simulink model "simplifiedModel"  (R2025b)
settings: Solver=VariableStepAuto  StartTime=0.0  StopTime=30  RelTol=1e-3
undefined symbols (not defined in the file or in its folder): aRef, CR_AR, CR_mC, CR_Plan, CR_pos, dRef, NFins, rocketLength, rT, SF_aFin, SF_AR, SF_CG, SF_CP_Sub, SF_CP_sup, SF_H, SF_mC, SF_plan, SF_RC, SF_TC, yMac
libraries: aerolibasang x3, aerolibanim x2, simulink_extras x1, aerolibatmos2 x1
settings Model: Creator=Ranvir  LastModifiedBy=Ranvir

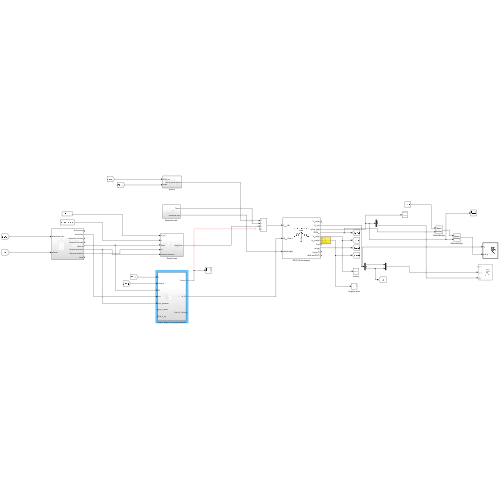
[thumbnail: Simulink's stored preview of the top-level diagram]
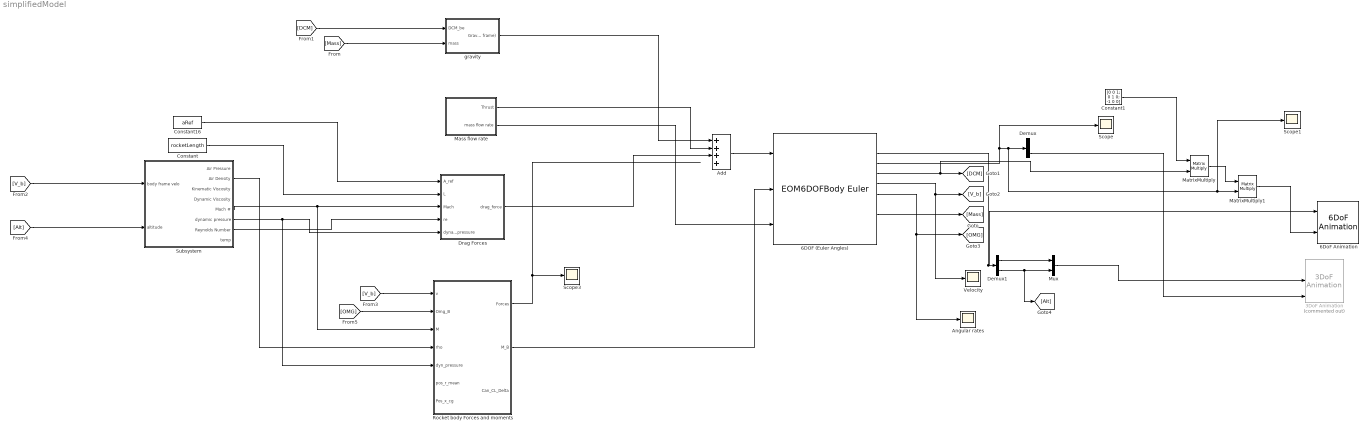
== system simplifiedModel ==
  3DoF Animation : aerolibanim/3DoF Animation  Commented=on  u1=[0 5000 -2000 2000 -5050 -3050]  u2=0.05  u3=10  u5=Fixed position  u6=[2000 500 -3150]  u7=10  u8=on
  6DOF (Euler Angles) : EOM6DOFBodyEuler  mtype=Simple Variable  eul_0=[0 deg2rad(5) 0]  mass_0=23.434  mass_e=16.5  mass_f=23.434  inertia_e=[9.947 0 0; 0 9.947 0; 0 0 0.14158]  inertia_f=[14.126568 0 0; 0 14.126568 0; 0 0 0.201075]  mass_flag=on
  6DoF Animation : aerolibanim/6DoF Animation  u1=[0 4000 -2000 2000 -5000 -3000]  u2=0.01  u3=100  u4=[4000 0 -5000]  u5=Fly alongside  u6=[2000 500 -3150]  u7=2  u8=off
  Add : Sum  Inputs=++++
  Angular rates : Scope
      settings: ActiveDisplayYMinimum=-0.094477943134186726  ActiveDisplayYMaximum=0.85030148820768081  DataLoggingVariableName=ScopeData8
  Constant : Constant  Value=rocketLength
  Constant1 : Constant  Value=[0 0 1; 0 1 0; -1 0 0]
  Constant16 : Constant  Value=aRef
  Demux : Demux  Outputs=3
  Demux1 : Demux  Outputs=3
  Drag Forces : Subsystem
  Mass flow rate : Subsystem
  MatrixMultiply : Product  Multiplication=Matrix(*)
  MatrixMultiply1 : Product  Multiplication=Matrix(*)
  Mux : Mux  Inputs=2
  Rocket body Forces and moments : Subsystem
  Scope : Scope
      settings: ActiveDisplayYMinimum=-3.9094785431209607  ActiveDisplayYMaximum=3.92160420988626
  Scope1 : Scope
      settings: ActiveDisplayYMinimum=-1  ActiveDisplayYMaximum=1  DataLoggingVariableName=ScopeData2
  Scope3 : Scope
      settings: ActiveDisplayYMinimum=-1.6641307477969988E+6  ActiveDisplayYMaximum=1.5617591567603932E+6  DataLoggingVariableName=ScopeData10
  Subsystem : Subsystem
  Velocity : Scope
      settings: ActiveDisplayYMinimum=-80.5453519654905  ActiveDisplayYMaximum=285.45576994763  DataLoggingVariableName=ScopeData11
  gravity : Subsystem
  wires:
  Subsystem/5(Mach #) -> Drag Forces/3(Mach), Rocket body Forces and moments/3(M)
  Subsystem/7(Reynolds Number) -> Drag Forces/4(re)
  Subsystem/6(dynamic pressure) -> Rocket body Forces and moments/5(dyn_pressure), Drag Forces/5(dynamic pressure)
  Constant16/1 -> Drag Forces/1(A_ref)
  Constant/1 -> Drag Forces/2(L)
  Mass flow rate/1(Thrust) -> Add/2
  gravity/1(Gravity (body frame)) -> Add/1
  Mass flow rate/2(mass flow rate) -> 6DOF (Euler Angles)/3
  6DOF (Euler Angles)/8 -> [Mass]
  [Mass] -> gravity/2(mass)
  6DOF (Euler Angles)/4 -> MatrixMultiply/2, [DCM]
  [DCM] -> gravity/1(DCM_be)
  Add/1 -> 6DOF (Euler Angles)/1
  Drag Forces/1(drag_force) -> Add/3
  Rocket body Forces and moments/2(M_B) -> 6DOF (Euler Angles)/2
  6DOF (Euler Angles)/3 -> Scope/1, Scope1/1, MatrixMultiply1/2, Demux/1
  6DOF (Euler Angles)/2 -> 6DoF Animation/1, Demux1/1
  Demux1/1 -> Mux/1
  Demux1/3 -> [Alt], Mux/2
  Mux/1 -> 3DoF Animation/2
  6DOF (Euler Angles)/5 -> Velocity/1, [V_b]
  [V_b] -> Subsystem/1(body frame velo)
  [V_b] -> Rocket body Forces and moments/1(v)
  6DOF (Euler Angles)/6 -> Angular rates/1, [OMG]
  [Alt] -> Subsystem/2(altitude)
  [OMG] -> Rocket body Forces and moments/2(Omg_B)
  Subsystem/2(Air Density) -> Rocket body Forces and moments/4(rho)
  Demux/3 -> 3DoF Animation/3
  Constant1/1 -> MatrixMultiply/1
  MatrixMultiply/1 -> MatrixMultiply1/1
  MatrixMultiply1/1 -> 6DoF Animation/2
  Rocket body Forces and moments/1(Forces) -> Scope3/1

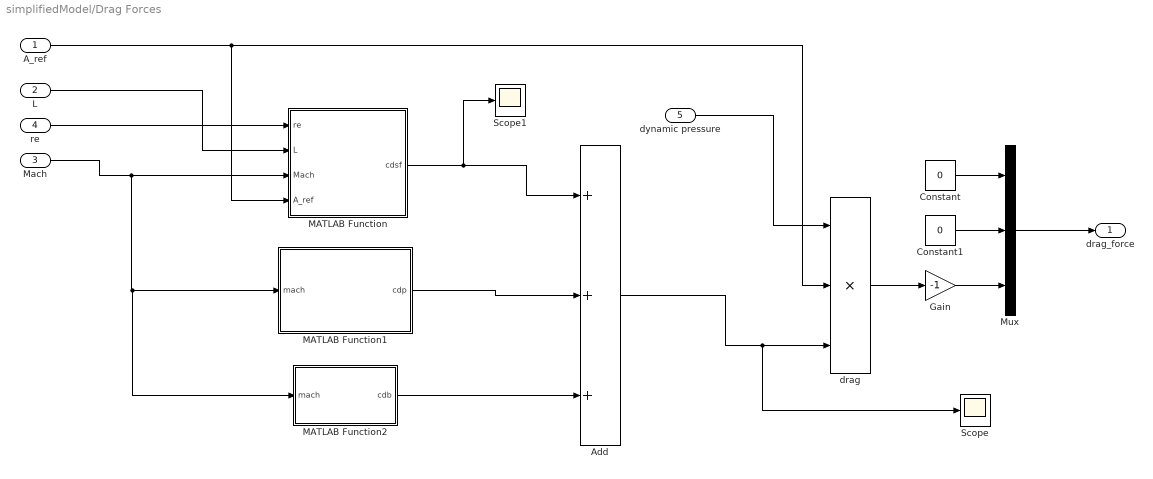
== system simplifiedModel/Drag Forces ==
  A_ref : Inport
  L : Inport  Port=2
  Mach : Inport  Port=3
  re : Inport  Port=4
  dynamic pressure : Inport  Port=5
  Add : Sum  Inputs=+++
  Constant : Constant  Value=0
  Constant1 : Constant  Value=0
  Gain : Gain  Gain=-1
  MATLAB Function : MATLAB Function  TreatAsAtomicUnit=on
  MATLAB Function1 : MATLAB Function  TreatAsAtomicUnit=on
  MATLAB Function2 : MATLAB Function  TreatAsAtomicUnit=on
  Mux : Mux  Inputs=3
  Scope : Scope
      settings: ActiveDisplayYMinimum=0.21944409933855474  ActiveDisplayYMaximum=1.41457657842317  DataLoggingVariableName=ScopeData7
  Scope1 : Scope
      settings: ActiveDisplayYMinimum=0.20880537476084277  ActiveDisplayYMaximum=1.0462233981932223  DataLoggingVariableName=ScopeData9
  drag : Product  Inputs=3
  drag_force : Outport
  wires:
  L/1 -> MATLAB Function/2(L)
  A_ref/1 -> drag/2, MATLAB Function/4(A_ref)
  Mach/1 -> MATLAB Function2/1(mach), MATLAB Function1/1(mach), MATLAB Function/3(Mach)
  re/1 -> MATLAB Function/1(re)
  MATLAB Function2/1(cdb) -> Add/3
  MATLAB Function1/1(cdp) -> Add/2
  MATLAB Function/1(cdsf) -> Scope1/1, Add/1
  dynamic pressure/1 -> drag/1
  Add/1 -> Scope/1, drag/3
  drag/1 -> Gain/1
  Mux/1 -> drag_force/1
  Constant1/1 -> Mux/2
  Gain/1 -> Mux/3
  Constant/1 -> Mux/1

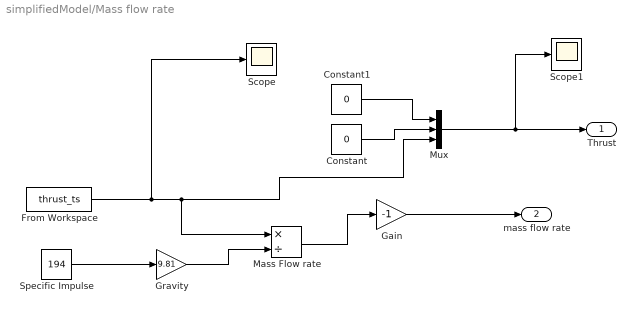
== system simplifiedModel/Mass flow rate ==
  Constant : Constant  Value=0
  Constant1 : Constant  Value=0
  From Workspace : FromWorkspace  VariableName=thrust_ts  OutputAfterFinalValue=Setting to zero
  Gain : Gain  Gain=-1
  Gravity : Gain  Gain=9.81
  Mass Flow rate : Product  Inputs=*/
  Mux : Mux  Inputs=3
  Scope : Scope
      settings: DataLoggingVariableName=ScopeData6
  Scope1 : Scope
      settings: ActiveDisplayYMinimum=-1  ActiveDisplayYMaximum=1
  Specific Impulse : Constant  Value=194
  Thrust : Outport
  mass flow rate : Outport  Port=2
  wires:
  Mass Flow rate/1 -> Gain/1
  Gravity/1 -> Mass Flow rate/2
  Specific Impulse/1 -> Gravity/1
  From Workspace/1 -> Scope/1, Mux/3, Mass Flow rate/1
  Gain/1 -> mass flow rate/1
  Constant/1 -> Mux/2
  Constant1/1 -> Mux/1
  Mux/1 -> Scope1/1, Thrust/1

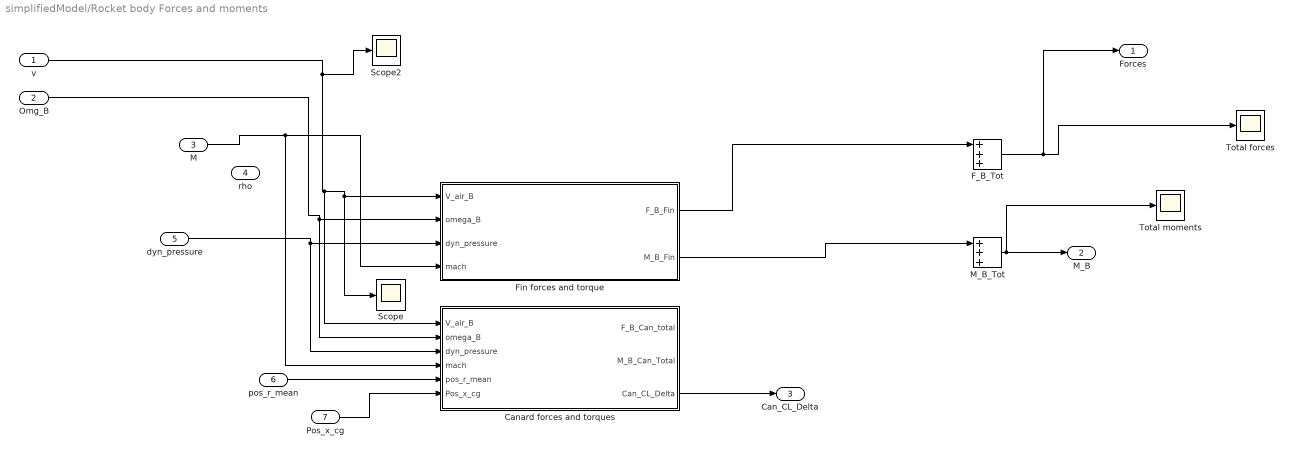
== system simplifiedModel/Rocket body Forces and moments ==
  v : Inport
  Omg_B : Inport  Port=2
  M : Inport  Port=3
  rho : Inport  Port=4
  dyn_pressure : Inport  Port=5
  pos_r_mean : Inport  Port=6
  Pos_x_cg : Inport  Port=7
  Canard forces and torques : Subsystem
  F_B_Tot : Sum  Inputs=+++
  Fin forces and torque : Subsystem
  M_B_Tot : Sum  Inputs=+++
  Scope : Scope
      settings: ActiveDisplayYMinimum=-0.018508285271356052  ActiveDisplayYMaximum=0.020281407753936571  DataLoggingVariableName=ScopeData15
  Scope2 : Scope
      settings: ActiveDisplayYMinimum=-769.59974570590657  ActiveDisplayYMaximum=2344.982620265816  DataLoggingVariableName=ScopeData16
  Total forces : Scope
      settings: ActiveDisplayYMinimum=-5.1479877420967748  ActiveDisplayYMaximum=7.0544525068547062  DataLoggingVariableName=ScopeData19
  Total moments : Scope
      settings: ActiveDisplayYMinimum=-0.69221418098949072  ActiveDisplayYMaximum=0.72914847927075177  DataLoggingVariableName=ScopeData17
  Forces : Outport
  M_B : Outport  Port=2
  Can_CL_Delta : Outport  Port=3
  wires:
  Fin forces and torque/1(F_B_Fin) -> F_B_Tot/1
  M_B_Tot/1 -> Total moments/1, M_B/1
  Canard forces and torques/3(Can_CL_Delta) -> Can_CL_Delta/1
  F_B_Tot/1 -> Forces/1, Total forces/1
  v/1 -> Canard forces and torques/1(V_air_B), Scope/1, Fin forces and torque/1(V_air_B), Scope2/1
  Omg_B/1 -> Canard forces and torques/2(omega_B), Fin forces and torque/2(omega_B)
  M/1 -> Canard forces and torques/4(mach), Fin forces and torque/4(mach)
  dyn_pressure/1 -> Canard forces and torques/3(dyn_pressure), Fin forces and torque/3(dyn_pressure)
  pos_r_mean/1 -> Canard forces and torques/5(pos_r_mean)
  Pos_x_cg/1 -> Canard forces and torques/6(Pos_x_cg)
  Fin forces and torque/2(M_B_Fin) -> M_B_Tot/1

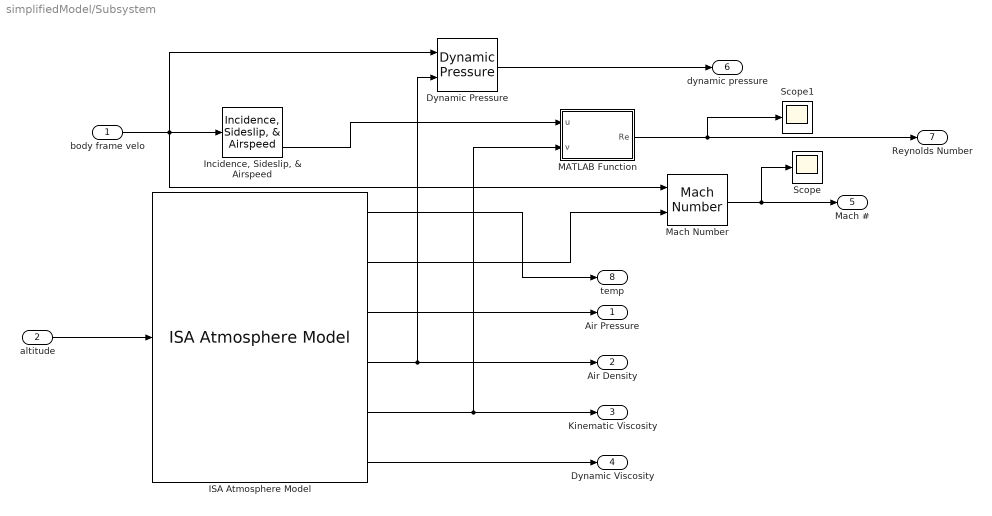
== system simplifiedModel/Subsystem ==
  body frame velo : Inport
  altitude : Inport  Port=2
  Dynamic Pressure : aerolibasang/Dynamic Pressure
  ISA Atmosphere Model : aerolibatmos2/ISA Atmosphere Model  useExtended=off  action=None  custom=off  viscosityOut=on  g=9.80665  gamma=1.4  R=287.0531  L=0.0065  h_trop=11000  h_strat=20000  rho0=1.225  P0=101325  T0=288.15  h0=0  S=110.4  Tref=273.15  muref=1.716e-5
  "Incidence, Sideslip, & Airspeed" : aerolibasang/Incidence, Sideslip, & Airspeed
  MATLAB Function : MATLAB Function  TreatAsAtomicUnit=on
  Mach Number : aerolibasang/Mach Number
  Scope : Scope
      settings: ActiveDisplayYMinimum=-1  ActiveDisplayYMaximum=1  DataLoggingVariableName=ScopeData4
  Scope1 : Scope
      settings: ActiveDisplayYMinimum=-4.9384528358794907E+6  ActiveDisplayYMaximum=4.4446075522915423E+7  DataLoggingVariableName=ScopeData5
  Air Pressure : Outport
  Air Density : Outport  Port=2
  Kinematic Viscosity : Outport  Port=3
  Dynamic Viscosity : Outport  Port=4
  Mach # : Outport  Port=5
  dynamic pressure : Outport  Port=6
  Reynolds Number : Outport  Port=7
  temp : Outport  Port=8
  wires:
  ISA Atmosphere Model/2 -> Mach Number/2
  ISA Atmosphere Model/5 -> MATLAB Function/2(v), Kinematic Viscosity/1
  ISA Atmosphere Model/4 -> Dynamic Pressure/2, Air Density/1
  ISA Atmosphere Model/3 -> Air Pressure/1
  ISA Atmosphere Model/6 -> Dynamic Viscosity/1
  Mach Number/1 -> Scope/1, Mach #/1
  altitude/1 -> ISA Atmosphere Model/1
  Dynamic Pressure/1 -> dynamic pressure/1
  body frame velo/1 -> Dynamic Pressure/1, Mach Number/1, "Incidence, Sideslip, & Airspeed"/1
  "Incidence, Sideslip, & Airspeed"/3 -> MATLAB Function/1(u)
  MATLAB Function/1(Re) -> Reynolds Number/1, Scope1/1
  ISA Atmosphere Model/1 -> temp/1

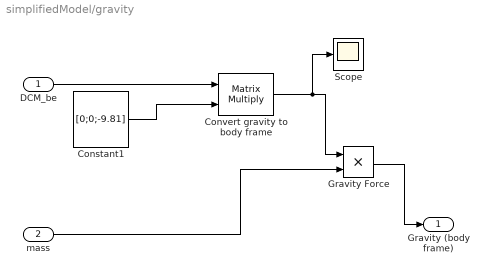
== system simplifiedModel/gravity ==
  DCM_be : Inport
  mass : Inport  Port=2
  Constant1 : Constant  Value=[0;0;-9.81]  VectorParams1D=off
  Convert gravity to body frame : Product  Multiplication=Matrix(*)
  Gravity Force : Product
  Scope : Scope
      settings: ActiveDisplayYMinimum=-1  ActiveDisplayYMaximum=1  DataLoggingVariableName=ScopeData3
  Gravity (body frame) : Outport
  wires:
  mass/1 -> Gravity Force/2
  Gravity Force/1 -> Gravity (body frame)/1
  Constant1/1 -> Convert gravity to body frame/2
  DCM_be/1 -> Convert gravity to body frame/1
  Convert gravity to body frame/1 -> Scope/1, Gravity Force/1

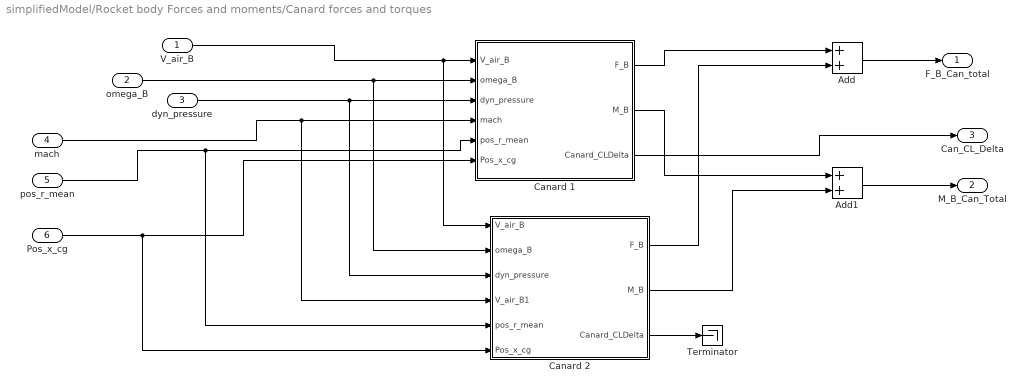
== system simplifiedModel/Rocket body Forces and moments/Canard forces and torques ==
  V_air_B : Inport
  omega_B : Inport  Port=2
  dyn_pressure : Inport  Port=3
  mach : Inport  Port=4
  pos_r_mean : Inport  Port=5
  Pos_x_cg : Inport  Port=6
  Add : Sum
  Add1 : Sum
  Canard 1 : Subsystem
  Canard 2 : Subsystem
  Terminator : Terminator
  F_B_Can_total : Outport
  M_B_Can_Total : Outport  Port=2
  Can_CL_Delta : Outport  Port=3
  wires:
  Canard 1/1(F_B) -> Add/1
  Canard 2/1(F_B) -> Add/2
  Canard 1/2(M_B) -> Add1/1
  Canard 2/2(M_B) -> Add1/2
  Add/1 -> F_B_Can_total/1
  Add1/1 -> M_B_Can_Total/1
  Canard 1/3(Canard_CLDelta) -> Can_CL_Delta/1
  Canard 2/3(Canard_CLDelta) -> Terminator/1
  V_air_B/1 -> Canard 2/1(V_air_B), Canard 1/1(V_air_B)
  omega_B/1 -> Canard 2/2(omega_B), Canard 1/2(omega_B)
  dyn_pressure/1 -> Canard 2/3(dyn_pressure), Canard 1/3(dyn_pressure)
  mach/1 -> Canard 2/4(V_air_B1), Canard 1/4(mach)
  pos_r_mean/1 -> Canard 2/5(pos_r_mean), Canard 1/5(pos_r_mean)
  Pos_x_cg/1 -> Canard 2/6(Pos_x_cg), Canard 1/6(Pos_x_cg)

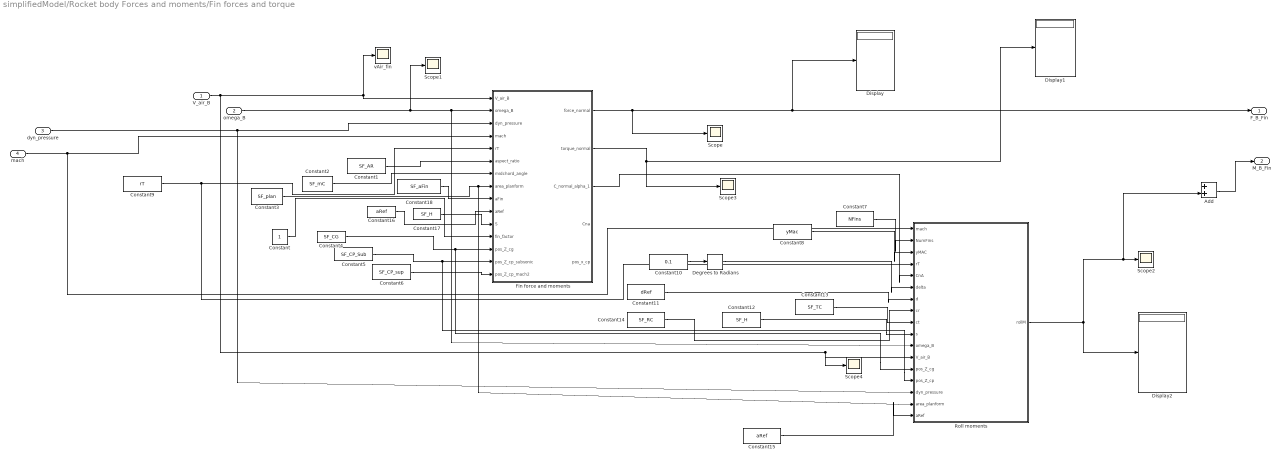
== system simplifiedModel/Rocket body Forces and moments/Fin forces and torque ==
  V_air_B : Inport
  omega_B : Inport  Port=2
  dyn_pressure : Inport  Port=3
  mach : Inport  Port=4
  Add : Sum
  Constant : Constant
  Constant1 : Constant  Value=SF_AR
  Constant10 : Constant  Value=0.1
  Constant11 : Constant  Value=dRef
  Constant12 : Constant  Value=SF_H
  Constant13 : Constant  Value=SF_TC
  Constant14 : Constant  Value=SF_RC
  Constant15 : Constant  Value=aRef
  Constant16 : Constant  Value=aRef
  Constant17 : Constant  Value=SF_H
  Constant18 : Constant  Value=SF_aFin
  Constant2 : Constant  Value=SF_mC
  Constant3 : Constant  Value=SF_plan
  Constant4 : Constant  Value=SF_CG
  Constant5 : Constant  Value=SF_CP_Sub
  Constant6 : Constant  Value=SF_CP_sup
  Constant7 : Constant  Value=NFins
  Constant8 : Constant  Value=yMac
  Constant9 : Constant  Value=rT
  Degrees to Radians : simulink_extras/Transformations/Degrees to Radians
  Display : Display
  Display1 : Display
  Display2 : Display
  Fin force and moments : MATLAB Function  TreatAsAtomicUnit=on
  Roll moments : MATLAB Function  TreatAsAtomicUnit=on
  Scope{,1..4} (5 alike) : Scope
      Scope settings: ActiveDisplayYMinimum=-38.327533693921524  ActiveDisplayYMaximum=344.94780324529376  DataLoggingVariableName=ScopeData13
      Scope1 settings: ActiveDisplayYMinimum=-1  ActiveDisplayYMaximum=1  DataLoggingVariableName=ScopeData23
      Scope2 settings: ActiveDisplayYMinimum=-0.01388327582792423  ActiveDisplayYMaximum=0.055054556987143094  DataLoggingVariableName=ScopeData24
      Scope3 settings: ActiveDisplayYMinimum=-1  ActiveDisplayYMaximum=1  DataLoggingVariableName=ScopeData27
      Scope4 settings: ActiveDisplayYMinimum=-1  ActiveDisplayYMaximum=1  DataLoggingVariableName=ScopeData28
  vAir_fin : Scope
      settings: ActiveDisplayYMinimum=-80.543649923632159  ActiveDisplayYMaximum=285.44044964997647  DataLoggingVariableName=ScopeData14
  F_B_Fin : Outport
  M_B_Fin : Outport  Port=2
  wires:
  Fin force and moments/1(force_normal) -> Scope/1, Display/1, F_B_Fin/1
  Fin force and moments/2(torque_normal) -> Scope3/1, Display1/1
  Constant6/1 -> Fin force and moments/15(pos_Z_cp_mach2)
  Constant5/1 -> Roll moments/14(pos_Z_cp), Fin force and moments/14(pos_Z_cp_subsonic)
  Constant4/1 -> Roll moments/13(pos_Z_cg), Fin force and moments/13(pos_Z_cg)
  Constant/1 -> Fin force and moments/12(fin_factor)
  Constant3/1 -> Roll moments/16(area_planform), Fin force and moments/8(area_planform)
  Constant2/1 -> Fin force and moments/7(midchord_angle)
  Constant1/1 -> Fin force and moments/6(aspect_ratio)
  V_air_B/1 -> Scope4/1, Roll moments/12(V_air_B), vAir_fin/1, Fin force and moments/1(V_air_B)
  mach/1 -> Roll moments/1(mach), Fin force and moments/4(mach)
  dyn_pressure/1 -> Roll moments/15(dyn_pressure), Fin force and moments/3(dyn_pressure)
  omega_B/1 -> Roll moments/11(omega_B), Fin force and moments/2(omega_B), Scope1/1
  Constant7/1 -> Roll moments/2(NumFins)
  Constant11/1 -> Roll moments/7(d)
  Constant10/1 -> Degrees to Radians/1
  Constant9/1 -> Roll moments/4(rT), Fin force and moments/5(rT)
  Constant8/1 -> Roll moments/3(yMAC)
  Constant12/1 -> Roll moments/10(s)
  Constant13/1 -> Roll moments/9(ct)
  Constant14/1 -> Roll moments/8(cr)
  Roll moments/1(rollM) -> Add/2, Scope2/1, Display2/1
  Constant15/1 -> Roll moments/17(aRef)
  Constant16/1 -> Fin force and moments/10(aRef)
  Constant17/1 -> Fin force and moments/11(S)
  Constant18/1 -> Fin force and moments/9(aFin)
  Degrees to Radians/1 -> Roll moments/6(delta)
  Fin force and moments/3(C_normal_alpha_1) -> Roll moments/5(CnA)
  Add/1 -> M_B_Fin/1

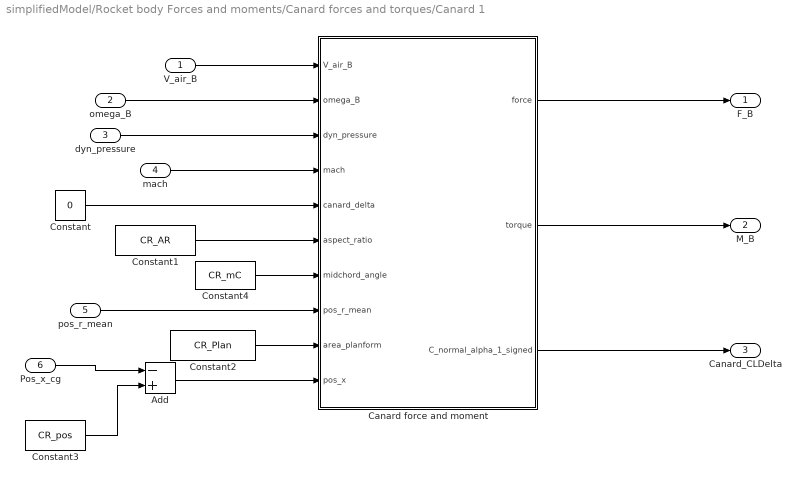
== system simplifiedModel/Rocket body Forces and moments/Canard forces and torques/Canard 1 ==
  V_air_B : Inport
  omega_B : Inport  Port=2
  dyn_pressure : Inport  Port=3
  mach : Inport  Port=4
  pos_r_mean : Inport  Port=5
  Pos_x_cg : Inport  Port=6
  Add : Sum  Inputs=-+
  Canard force and moment : MATLAB Function  TreatAsAtomicUnit=on
  Constant : Constant  Value=0
  Constant1 : Constant  Value=CR_AR
  Constant2 : Constant  Value=CR_Plan
  Constant3 : Constant  Value=CR_pos
  Constant4 : Constant  Value=CR_mC
  F_B : Outport
  M_B : Outport  Port=2
  Canard_CLDelta : Outport  Port=3
  wires:
  Canard force and moment/1(force) -> F_B/1
  Canard force and moment/2(torque) -> M_B/1
  Canard force and moment/3(C_normal_alpha_1_signed) -> Canard_CLDelta/1
  Constant/1 -> Canard force and moment/5(canard_delta)
  V_air_B/1 -> Canard force and moment/1(V_air_B)
  omega_B/1 -> Canard force and moment/2(omega_B)
  dyn_pressure/1 -> Canard force and moment/3(dyn_pressure)
  mach/1 -> Canard force and moment/4(mach)
  pos_r_mean/1 -> Canard force and moment/8(pos_r_mean)
  Pos_x_cg/1 -> Add/1
  Add/1 -> Canard force and moment/10(pos_x)
  Constant3/1 -> Add/2
  Constant2/1 -> Canard force and moment/9(area_planform)
  Constant1/1 -> Canard force and moment/6(aspect_ratio)
  Constant4/1 -> Canard force and moment/7(midchord_angle)

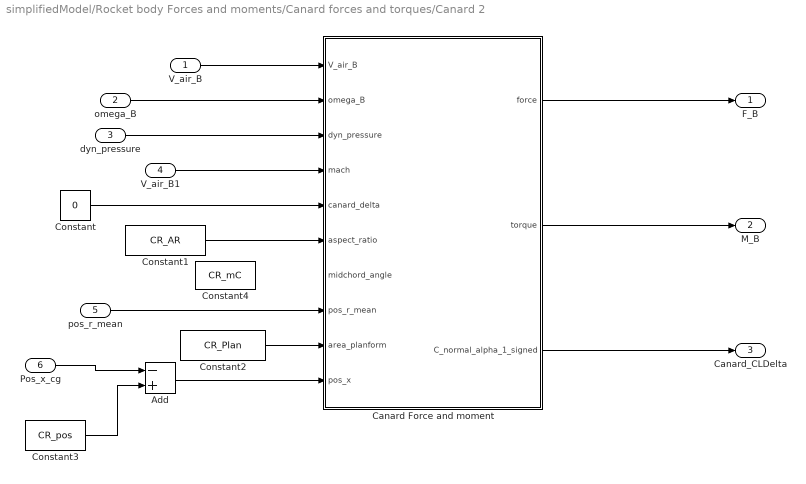
== system simplifiedModel/Rocket body Forces and moments/Canard forces and torques/Canard 2 ==
  V_air_B : Inport
  omega_B : Inport  Port=2
  dyn_pressure : Inport  Port=3
  V_air_B1 : Inport  Port=4
  pos_r_mean : Inport  Port=5
  Pos_x_cg : Inport  Port=6
  Add : Sum  Inputs=-+
  Canard Force and moment : MATLAB Function  TreatAsAtomicUnit=on
  Constant : Constant  Value=0
  Constant1 : Constant  Value=CR_AR
  Constant2 : Constant  Value=CR_Plan
  Constant3 : Constant  Value=CR_pos
  Constant4 : Constant  Value=CR_mC
  F_B : Outport
  M_B : Outport  Port=2
  Canard_CLDelta : Outport  Port=3
  wires:
  Canard Force and moment/1(force) -> F_B/1
  Canard Force and moment/2(torque) -> M_B/1
  Canard Force and moment/3(C_normal_alpha_1_signed) -> Canard_CLDelta/1
  V_air_B1/1 -> Canard Force and moment/4(mach)
  omega_B/1 -> Canard Force and moment/2(omega_B)
  Constant2/1 -> Canard Force and moment/9(area_planform)
  V_air_B/1 -> Canard Force and moment/1(V_air_B)
  dyn_pressure/1 -> Canard Force and moment/3(dyn_pressure)
  Constant/1 -> Canard Force and moment/5(canard_delta)
  Constant3/1 -> Add/2
  Pos_x_cg/1 -> Add/1
  Constant1/1 -> Canard Force and moment/6(aspect_ratio)
  pos_r_mean/1 -> Canard Force and moment/8(pos_r_mean)
  Add/1 -> Canard Force and moment/10(pos_x)

== matlab function simplifiedModel/Rocket body Forces and moments/Fin forces and torque/Roll moments ==
  data: mach input; NumFins input; rollM output; yMAC input; rT input; CnA input; delta input; d input; cr input; ct input; s input; omega_B input; V_air_B input; pos_Z_cg input; pos_Z_cp input; dyn_pressure input; area_planform input; aRef input
function rollM  = roll_moment(mach, NumFins, yMAC, rT, CnA, delta, d, cr, ct,s, omega_B, V_air_B, pos_Z_cg, pos_Z_cp, dyn_pressure, area_planform, aRef)
    



   
    pos_z = (pos_Z_cp - pos_Z_cg) * [0;0;1];
    
    % need to know incidence angle and how to convert vector into direciton
    %%% relative velocity


    %Define the vector using the wind vector, use that to create the moment
    %definition (z axis in the body frame) then multiply that with the 
    
    %%% relative velocity
    Vrel = V_air_B + cross(omega_B, pos_z);

    
    Vrel_Z = Vrel(3);
    Vrel_mag = norm(Vrel);
   
    beta = sqrt(abs(1-mach^2));
    cn_0 = (2*pi)/beta;


    rollForcing = (NumFins*(yMAC+rT)*CnA*delta)/s;
    %% Roll damping bs
    if Vrel(3) ~= 0
        %sumTerm = (((cr+ct)/2)*(rT^2)*s) + (((cr+(2*ct))/3)*(s^2)*rT) + (((cr+(3*ct))/12)*(s^3));
    
        %Fix from chatgpt
        sumTerm = ((cr+ct)/2)      * (rT^2) * s  + ...
          ((cr+2*ct)/3)    * (rT)   * (s^2) + ...
          ((cr+3*ct)/12)   * (s^3);

        rDampCoeff = ((NumFins*cn_0*omega_B(3))/(aRef*d*Vrel_mag))*sumTerm

    
            
        cRl = rollForcing - rDampCoeff;
    
        F_N_dir = [
                   0;
                   0;
                   Vrel_Z/Vrel_mag;
                  ];
        
         f_m = cRl * dyn_pressure * aRef*d;

         rollM = [0; 0; f_m;];
    else
        rollM =[0; 0; 0;];
 
    %rollM = cross(pos_z, force_normal);

end

== matlab function simplifiedModel/Rocket body Forces and moments/Canard forces and torques/Canard 1/Canard force and moment ==
  data: V_air_B input; force output; omega_B input; dyn_pressure input; mach input; canard_delta input; aspect_ratio input; midchord_angle input; pos_r_mean input; area_planform input; pos_x input; torque output; C_normal_alpha_1_signed output
function [force, torque, C_normal_alpha_1_signed] = canard_dynamics(V_air_B, omega_B, dyn_pressure, mach, canard_delta, aspect_ratio, midchord_angle, pos_r_mean, area_planform, pos_x)
    % canard position
    pos = [pos_x; pos_r_mean; 0];

    % relative velocity
    Vrel = V_air_B + cross(omega_B, pos);
    
    % local incidence 
    alpha_local = atan2(Vrel(3), Vrel(1));
    incidence = canard_delta - alpha_local;
    
    % calculate coefficient of planar surface
    C_normal_alpha_1 = aerosurface_calc(mach, incidence, aspect_ratio, midchord_angle);
    C_normal_alpha_1_signed = C_normal_alpha_1 * sign(Vrel(1));
    
    % force and torque
    force = C_normal_alpha_1 * area_planform * sin(incidence) * dyn_pressure * [0; 0; 1];
    torque = cross(pos, force);
end

== matlab function simplifiedModel/Drag Forces/MATLAB Function ==
  data: re input; L input; cdsf output; Mach input; A_ref input
function cdsf = skin_friction(re,L, Mach,A_ref)

r_s = 425e-6;

f_b = 8.93;
chord_mean = 0.23456;
t = 0.00686;

A_wetbody = 0.7009;
A_wetfin = 0.1609;

re_crit = 51*(r_s/L)^-1.039;

if re < 10^4
    cf = 1.48e-2;
elseif re >= 10^4 && re < re_crit
    cf = 1 / (1.5*log(re) - 5.6)^2;
else
    cf = 0.032*(r_s/L)^0.2;
end

if Mach < 1
    c_fc = cf*(1-0.1*Mach^2);
else 
    c_fc = cf/(1+0.15*Mach^2)^0.58;
end

cdsf = c_fc * (((1+(1/(2*f_b)))*A_wetbody + ((1+(2*t/chord_mean)))*A_wetfin)/A_ref);

== matlab function simplifiedModel/Subsystem/MATLAB Function ==
  data: u input; Re output; v input
function Re = reynolds(u,v)
L = 2.13;

Re = (u*L)/v;

== matlab function simplifiedModel/Drag Forces/MATLAB Function1 ==
  data: cdp output; mach input
function cdp = pressure_drag(mach)

sweep_angle = 1.13446;

if mach < 0.9
    cd_le = (1-mach^2)^(-0.417) - 1;
elseif mach>=0.9 && mach<1
   cd_le = 1-1.785*(mach-0.9);
else
    cd_le = 1.214-((0.502)/(mach^2))+((0.1095)/(mach^4));
end

cdp = cd_le * cos(sweep_angle)^2;

== matlab function simplifiedModel/Drag Forces/MATLAB Function2 ==
  data: mach input; cdb output
function cdb = base_drag(mach)

if mach < 1
    cdb = 0.12 + 0.13*mach^2;
else
    cdb = 0.25/mach;
end

== matlab function simplifiedModel/Rocket body Forces and moments/Fin forces and torque/Fin force and moments ==
  data: V_air_B input; force_normal output; omega_B input; dyn_pressure input; mach input; rT input; aspect_ratio input; midchord_angle input; area_planform input; aFin input; aRef input; S input; fin_factor input; pos_Z_cg input; pos_Z_cp_subsonic input; pos_Z_cp_mach2 input; torque_normal output; C_normal_alpha_1 output; Cna output; pos_x_cp output
function [force_normal, torque_normal, C_normal_alpha_1, Cna,  pos_x_cp] = fin_dynamics(V_air_B, omega_B, dyn_pressure, mach, rT, aspect_ratio, midchord_angle, area_planform, aFin, aRef, S, fin_factor, pos_Z_cg, pos_Z_cp_subsonic, pos_Z_cp_mach2)
 %%% Center of Pressure
    % threshold values
    subsonic = 0.8;
    supersonic = 1.6;

    % linear interpolation (for now)
    if mach <= subsonic
        pos_x_cp = pos_Z_cp_subsonic;
    elseif mach >= supersonic 
        pos_x_cp = pos_Z_cp_mach2;
    else % transonic
        pos_x_cp = (mach - supersonic) * (pos_Z_cp_subsonic - pos_Z_cp_mach2) / (subsonic - supersonic) + pos_Z_cp_mach2;
    end

    pos_z = (pos_x_cp - pos_Z_cg) * [0;0;1];

    
    %%% relative velocity
    Vrel = V_air_B + cross(omega_B, pos_z);

    % Body relative velocity magnitude
    Vrel_mag = norm(Vrel);
    Vrel_Z = Vrel(3);
    Vrel_magXY = norm(Vrel(1:2));
    incidence = atan2(Vrel_magXY,Vrel_Z);

    %%% calculate normal force coefficient
    C_normal_alpha_1 = aerosurface_calc(mach, incidence, aspect_ratio, midchord_angle)*(1+(rT/(S+rT)));
    
    Cna = (2*C_normal_alpha_1);
    %%% Forces
    if Vrel_magXY ~= 0 % prevent division by 0
        % Angle of attack and component separation
        
        F_N_dir = [
                   Vrel(1) / Vrel_magXY; 
                   Vrel(2) / Vrel_magXY;
                   0;
                  ];
        
        % Calculating total force
        F_N_mag = Cna * fin_factor * dyn_pressure * area_planform * sin(incidence);
        force_normal = F_N_dir * F_N_mag;
    else
        
        force_normal = [0; 0; 0];
    end

    % Total torque
    torque_normal = cross(pos_z, force_normal);
end

== matlab function simplifiedModel/Rocket body Forces and moments/Canard forces and torques/Canard 2/Canard Force and moment ==
  data: V_air_B input; force output; omega_B input; dyn_pressure input; mach input; canard_delta input; aspect_ratio input; midchord_angle input; pos_r_mean input; area_planform input; pos_x input; torque output; C_normal_alpha_1_signed output
function [force, torque, C_normal_alpha_1_signed] = canard_dynamics(V_air_B, omega_B, dyn_pressure, mach, canard_delta, aspect_ratio, midchord_angle, pos_r_mean, area_planform, pos_x)
    % canard position
    pos = [pos_x; pos_r_mean; 0];

    % relative velocity
    Vrel = V_air_B + cross(omega_B, pos);
    
    % local incidence 
    alpha_local = atan2(Vrel(3), Vrel(1));
    incidence = canard_delta - alpha_local;
    
    % calculate coefficient of planar surface
    C_normal_alpha_1 = aerosurface_calc(mach, incidence, aspect_ratio, midchord_angle);
    C_normal_alpha_1_signed = C_normal_alpha_1 * sign(Vrel(1));
    
    % force and torque
    force = C_normal_alpha_1 * area_planform * sin(incidence) * dyn_pressure * [0; 0; 1];
    torque = cross(pos, force);
end
